simulink model "Thermoelectric_model"  (R2019a)
settings: Solver=VariableStepAuto  StartTime=0.0  StopTime=10.0  RelTol=1e-3
settings Model: Creator=student  LastModifiedBy=Nolan

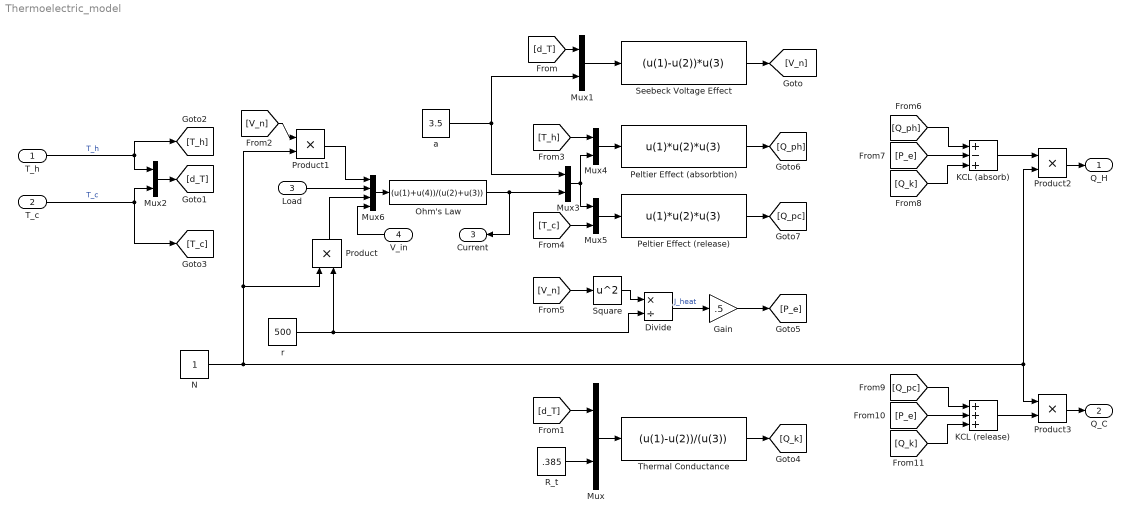
== system Thermoelectric_model ==
  T_h : Inport
  T_c : Inport  Port=2
  Load : Inport  Port=3
  "V_in " : Inport  Port=4
  Divide : Product  Inputs=*/
  Gain : Gain  Gain=.5
  KCL (absorb) : Sum  Inputs=+-+
  KCL (release) : Sum  Inputs=+++
  Mux{,1..5} (6 alike) : Mux  Inputs=2
  Mux6 : Mux
  N : Constant
  Ohm's Law : Fcn  Expr=(u(1)+u(4))/(u(2)+u(3))
  Peltier Effect (absorbtion) : Fcn  Expr=u(1)*u(2)*u(3)
  Peltier Effect (release) : Fcn  Expr=u(1)*u(2)*u(3)
  Product{,1..3} (4 alike) : Product
  "R_t " : Constant  Value=.385
  Seebeck Voltage Effect : Fcn  Expr=(u(1)-u(2))*u(3)
  Square : Math  Operator=square  SaturateOnIntegerOverflow=on
  Thermal Conductance : Fcn  Expr=(u(1)-u(2))/(u(3))
  a : Constant  Value=3.5
  r : Constant  Value=500
  Q_H : Outport  VectorParamsAs1DForOutWhenUnconnected=off
  Q_C : Outport  Port=2  VectorParamsAs1DForOutWhenUnconnected=off
  Current : Outport  Port=3  VectorParamsAs1DForOutWhenUnconnected=off
  wires:
  Mux/1 -> Thermal Conductance/1
  "R_t "/1 -> Mux/2
  Mux1/1 -> Seebeck Voltage Effect/1
  a/1 -> Mux1/2, Mux3/1
  Square/1 -> Divide/1
  r/1 -> Product/2, Divide/2
  T_h/1 -> [T_h], Mux2/1  "T_h"
  T_c/1 -> Mux2/2, [T_c]  "T_c"
  Mux4/1 -> Peltier Effect (absorbtion)/1
  Mux5/1 -> Peltier Effect (release)/1
  Ohm's Law/1 -> Mux3/2, Current/1
  Mux3/1 -> Mux5/1, Mux4/2
  Mux6/1 -> Ohm's Law/1
  Load/1 -> Mux6/2
  "V_in "/1 -> Mux6/4
  Product/1 -> Mux6/3
  Product1/1 -> Mux6/1
  N/1 -> Product2/2, Product3/1, Product1/2, Product/1
  Product2/1 -> Q_H/1
  KCL (absorb)/1 -> Product2/1
  KCL (release)/1 -> Product3/2
  Product3/1 -> Q_C/1
  Seebeck Voltage Effect/1 -> [V_n]
  Mux2/1 -> [d_T]
  [d_T] -> Mux1/1
  [d_T] -> Mux/1
  Thermal Conductance/1 -> [Q_k]
  Divide/1 -> Gain/1  "J_heat"
  Gain/1 -> [P_e]
  Peltier Effect (absorbtion)/1 -> [Q_ph]
  Peltier Effect (release)/1 -> [Q_pc]
  [V_n] -> Product1/1
  [T_h] -> Mux4/1
  [T_c] -> Mux5/2
  [V_n] -> Square/1
  [P_e] -> KCL (absorb)/2
  [Q_ph] -> KCL (absorb)/1
  [Q_k] -> KCL (absorb)/3
  [Q_pc] -> KCL (release)/1
  [P_e] -> KCL (release)/2
  [Q_k] -> KCL (release)/3
